simulink model "CML_Static_Sensory_Weighting"  (R2015a)
settings: Solver=ode4  SolverMode=MultiTasking  StartTime=0.0  StopTime=inf  FixedStep=BKIN_STEP_TIME  RelTol=1e-3
StartFcn:
  |  warndlg('Dexterit-E models cannot run under simulation. Please compile your model and run it from within Dexterit-E.');set_param(bdroot,'SimulationCommand','stop')
model workspace (MAT data in the model file):
  col_x = 1
  col_y = 2
  RADIUS_VIS = 3
  DELAY_POST_TRIAL_COL = 14
  BKIN_STEP_TIME = 0.00025
  START_WAIT_TIME_COL = 8
  E_START_TRIAL = 2
  E_START_REACHED = 4
  E_GO_CUE = 14
  E_MOVE_TIMEOUT = 21
  E_END_TRIAL = 20
  STROKE_WIDTH = 5
  K_HOLDTIME = 2
  K_ROBOT_RAMP_TIME = 3
  E_ROBOT_RETURN_TO_START = 10
  E_ENABLED_CONTROLLER = 31
  K_TIME_TO_START = 4
  E_HOLD_POS = 12
  BKIN_KINEMATIC_FRAME_SIZE = 400
  E_NO_EVENT = 0
  CP1 = 15
  CP2 = 16
  CP3 = 17
  CP4 = 18
  MOVE_TO_REF_TIME = 9
  REPOSITION_TIME = 11
  TRIAL_TYPE = 1
  E_RESPONSE_RECORDED = 18
  REPORT_TIME = 13
  REF_COLOR = 4
  START_TARGET_COL = 2
  REF_TARGET_COL = 3
  REF_HOLD_TIME = 10
  WAIT_REPORT_TIME = 12
  K_VEL_MIN = 1
  E_HAND_MOVING = 16
  E_MOVING_TO_REF = 6
  E_WAIT_AT_REF = 8
  TEXT1 = 6
  TEXT2 = 7
  TEXT3 = 8
  K_CUE_TARGET = 5
  E_START_REACHED2 = 5
  TEXT4 = 9
  CONTINUE = 4
  E_PAUSE = 40
  K_XJITTER = 6
  K_YJITTER = 7
  K_REF_START_TARGET = 8
  VY_TARG_OFFSET = 4
  PY_TARG_OFFSET = 5
  VX_TARG_OFFSET = 6
  PX_TARG_OFFSET = 7
libraries: Video x8, slrtlib x4, General x3, KINARM_general x2, KINARM_loads x2, xpcnilib x1
CloseFcn:
  | rtwprivate ssgencode ModelCloseRequest b2lab2d
settings Model: ModifiedComment=chris -- Wed Feb 16 09:18:30 2005 -- Version 1.1384  ModifiedHistory=Feb 16/05 - Add error repeat, add offset ramp  ExtModeArmWhenConnect=off  ExtModeLogAll=off  Creator=Chris Grebeldinger  LastModifiedBy=User
settings SolverCC: EnableConcurrentExecution=on  AutoInsertRateTranBlk=on
settings DataIOCC: LimitDataPoints=off  SignalLoggingSaveFormat=ModelDataLogs  SaveOutput=off  SaveTime=off  SignalLoggingName=sigsOut
settings OptimizationCC: BlockReduction=off  BooleanDataType=off  OptimizeBlockIOStorage=off  BufferReuse=off  GlobalBufferReuse=off  ExpressionFolding=off  ExpressionDepthLimit=2147483647  LocalBlockOutputs=off  InitFltsAndDblsToZero=on
settings DebuggingCC: SaveWithParameterizedLinksMsg=none  UnderspecifiedInitializationDetection=Classic  MergeDetectMultiDrivingBlocksExec=none  SignalResolutionControl=TryResolveAllWithWarning  MultiTaskDSMMsg=warning  FcnCallInpInsideContextMsg=UseLocalSettings  StateNameClashWarn=warning  StrictBusMsg=ErrorOnBusTreatedAsVector
settings HardwareCC: ProdIntDivRoundTo=Zero  ProdEndianess=LittleEndian  ProdLongLongMode=on  ProdHWDeviceType=Generic->32-bit x86 compatible  TargetHWDeviceType=32-bit Generic
settings SFSimCC: SimCustomHeaderCode="#include \"stdlib.h\""  SFSimEcho=off  SimParseCustomCode=off
settings RTWCC: SystemTargetFile=slrt.tlc  TemplateMakefile=slrt_default_tmf  Description=Simulink Real-Time  CustomSourceCode="#include \"stdlib.h\""
settings CodeAppCC: MaxIdLength=63
settings SimulinkRealTimeCC: TargetFcnLib=ansi_tfl_tmw.mat  GeneratePreprocessorConditionals=Disable all  xPCisDownloadable=off  xPCisDefaultEnv=off

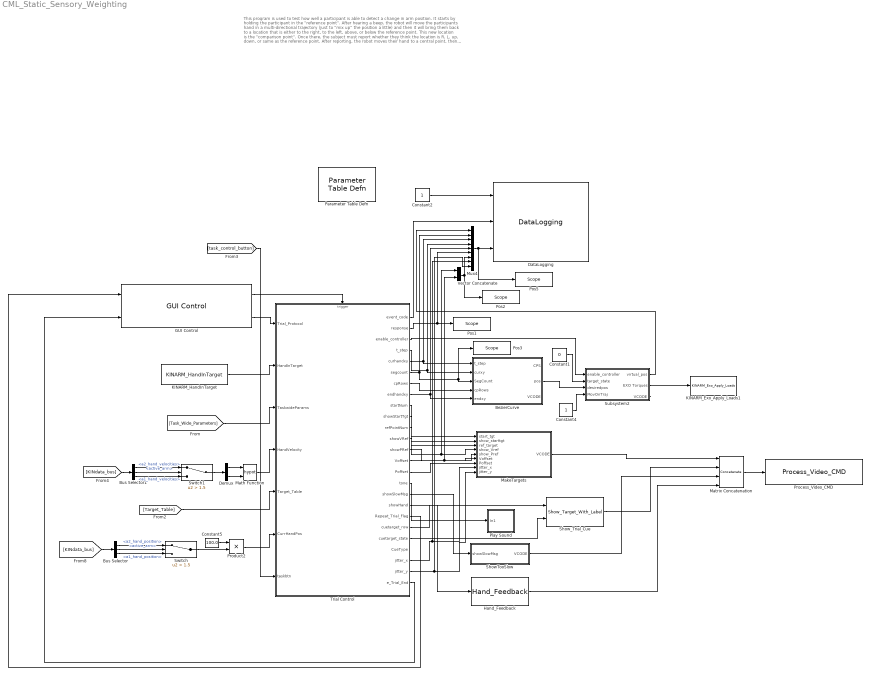
== system CML_Static_Sensory_Weighting ==
  note: This program is used to test how well a participant is able to detect a change in arm position.
      | It starts by holding the participant in the "reference point". After hearing a beep, the robot
      | will move the participants hand in a multi-directional trajectory (just to "mix up" the position a little)
      | and then it will bring them back to a location that is either to the right, to the left, above, or below
      | the reference point. This new location is the "comparison point". Once there, the subject must
      | report whether they think the location is R, L, up, down, or same as the reference point. After
      | reporting, the robot moves their hand to a central point, then back to the reference point to begin
      | the next trial.
      | A staircase updates for each direction, until a direction's staircase experiences 3 duirection
      | reversals in 6 trials, or 25 repetitions.
  BezierCurve : Subsystem
  Bus Selector : BusSelector  OutputSignals=Robot2.a2_hand_position,KINDataGeneral.active_arm,Robot1.a1_hand_position
  Bus Selector1 : BusSelector  OutputSignals=Robot2.a2_hand_velocities,KINDataGeneral.active_arm,Robot1.a1_hand_velocities
  Constant1 : Constant  Value=0
  Constant2 : Constant
  Constant4 : Constant
  Constant5 : Constant  Value=100.0
  DataLogging : General/DataLogging  log_event_codes=on  log_analog_inputs=on  show_time_remaining=off  ecat_include=on
  Demux : Demux  Outputs=2
  GUI Control : General/GUI Control  task_version=1.0  show_repeat_trial_flag=on  use_custom_tp=off  target_type_str=Circle  Target_Type=1  XYcols=[1 2]  Vcols=3  Lcols=4  indices_padding=[0 0 0 0;0 0 0 0]  target_table_rows=64  load_table_rows=20  tp_table_rows=100
  Hand_Feedback : KINARM_general/Hand_Feedback  feedback_cntl_src=status only
  KINARM_Exo_Apply_Loads1 : KINARM_loads/KINARM_Exo_Apply_Loads  up_duration=500  down_duration=500  max_torque=8  limit_motors=off
  KINARM_HandInTarget : KINARM_general/KINARM_HandInTarget  use_dominant_hand=on  target_type=Circle  num_states=1  attribcol1=[RADIUS_VIS]  attribcol2=[0]  attribcol3=[0]  attribcol4=[0]  attribcol5=[0]
  MakeTargets : Subsystem
  Math Function : Math  Operator=hypot  SaturateOnIntegerOverflow=on
  Matrix Concatenation : Concatenate  NumInputs=4  Mode=Multidimensional array
  Mux4 : Mux  Inputs=9
  Parameter Table Defn : General/Parameter Table Defn  ShowInLibBrowser=0
  Play Sound : Subsystem
  Pos1 : slrtlib/Displays and Logging/Scope   scopeno=2  scopetype=Target  autostart=on  viewmode=Numerical  formatstr='%15.6f'  grid=on  ylimits=[-10,10]  nosamples=250  noprepostsamples=0  interleave=1  triggermode=FreeRun  triggersignal=1  trigsignalfromport=off  triggerlevel=0.0  triggerslope=Either  triggerscope=1  triggersample=0  filename=data.dat  mode=Lazy  writesize=512  autorestart=off  dynamicfilemode=off  maxwritefilesize=512*1024^2
  Pos2 : slrtlib/Displays and Logging/Scope   scopeno=3  scopetype=Target  autostart=on  viewmode=Numerical  formatstr='%15.6f'  grid=on  ylimits=[-10,10]  nosamples=250  noprepostsamples=0  interleave=1  triggermode=FreeRun  triggersignal=1  trigsignalfromport=off  triggerlevel=0.0  triggerslope=Either  triggerscope=1  triggersample=0  filename=data.dat  mode=Lazy  writesize=512  autorestart=off  dynamicfilemode=off  maxwritefilesize=512*1024^2
  Pos3 : slrtlib/Displays and Logging/Scope   scopeno=4  scopetype=Target  autostart=on  viewmode=Numerical  formatstr='%15.6f'  grid=on  ylimits=[-10,10]  nosamples=250  noprepostsamples=0  interleave=1  triggermode=FreeRun  triggersignal=1  trigsignalfromport=off  triggerlevel=0.0  triggerslope=Either  triggerscope=1  triggersample=0  filename=data.dat  mode=Lazy  writesize=512  autorestart=off  dynamicfilemode=off  maxwritefilesize=512*1024^2
  Pos5 : slrtlib/Displays and Logging/Scope   scopeno=1  scopetype=Target  autostart=on  viewmode=Numerical  formatstr='%15.6f'  grid=on  ylimits=[-10,10]  nosamples=250  noprepostsamples=0  interleave=1  triggermode=FreeRun  triggersignal=1  trigsignalfromport=off  triggerlevel=0.0  triggerslope=Either  triggerscope=1  triggersample=0  filename=data.dat  mode=Lazy  writesize=512  autorestart=off  dynamicfilemode=off  maxwritefilesize=512*1024^2
  Process_Video_CMD : Video/Process_Video_CMD  video_delay=50
  Product2 : Product
  ShowTooSlow : Subsystem
  Show_Trial_Cue : Video/Show_Target_With_Label  target_type=Circle  num_states=4  attribcol1=[0 0 0 RADIUS_VIS TEXT1 REF_COLOR STROKE_WIDTH]  attribcol2=[0 0 0 RADIUS_VIS TEXT2 REF_COLOR STROKE_WIDTH]  attribcol3=[0 0 0 RADIUS_VIS TEXT3 REF_COLOR STROKE_WIDTH]  attribcol4=[0 0 0 RADIUS_VIS TEXT4 REF_COLOR STROKE_WIDTH]  attribcol5=[0 0 0 0 0 0 0]  stateindices_padding=[0 0 0 0;0 0 0 0;0 0 0 0;0 0 0 0;0 0 0 0]  source=dialog  opacity=100  target_display=Both subject and operator displays
  Subsystem2 : Subsystem
  Switch : Switch  Criteria=u2 > Threshold  Threshold=1.5
  Switch1 : Switch  Criteria=u2 > Threshold  Threshold=1.5
  Trial Control : Stateflow chart  TreatAsAtomicUnit=on
  Vector Concatenate : Concatenate
  wires:
  [Task_Wide_Parameters] -> Trial Control/3(TaskwideParams)
  Trial Control/1(event_code) -> DataLogging/2
  [KINdata_bus] -> Bus Selector1/1
  GUI Control/2 -> Trial Control/1(Trial_Protocol)
  Trial Control/7(cpRows) -> BezierCurve/4(cpRows)
  Trial Control/5(curhandxy) -> Mux4/4, BezierCurve/2(curxy)
  Trial Control/6(segcount) -> Pos3/1, BezierCurve/3(SegCount), Mux4/2
  Trial Control/4(t_step) -> BezierCurve/1(t_step), Mux4/3
  Trial Control/11(refPointNum) -> MakeTargets/3(ref_target)
  BezierCurve/2(pos) -> Subsystem2/3(desiredpos)
  KINARM_HandInTarget/1 -> Trial Control/2(HandInTarget)
  Trial Control/8(endhandxy) -> BezierCurve/5("endxy "), Mux4/5
  Trial Control/16(tone) -> Play Sound/1(In1)
  [Target_Table] -> Trial Control/5(Target_Table)
  Trial Control/19(Repeat_Trial_Flag) -> GUI Control/1
  Mux4/1 -> Pos5/1, DataLogging/3
  Constant2/1 -> DataLogging/1
  Subsystem2/2(EXO Torques) -> KINARM_Exo_Apply_Loads1/1
  Trial Control/25(e_Trial_End) -> GUI Control/2
  Subsystem2/3(VCODE) -> ?
  Subsystem2/1(virtual_pos) -> Mux4/1
  Constant4/1 -> Subsystem2/4(MovOnTraj)
  Trial Control/3(enable_controller) -> Subsystem2/1(enable_controller)
  [KINdata_bus] -> Bus Selector/1
  Bus Selector/2 -> Switch/2  "<active_arm>"
  Bus Selector/1 -> Switch/1  "<a2_hand_position>"
  Bus Selector/3 -> Switch/3  "<a1_hand_position>"
  Switch/1 -> Product2/2
  Constant5/1 -> Product2/1
  Product2/1 -> Trial Control/6(CurrHandPos)
  MakeTargets/1(VCODE) -> Matrix Concatenation/1
  Trial Control/2(response) -> Mux4/6, Pos1/1
  Trial Control/18(showHand) -> Hand_Feedback/1
  Hand_Feedback/1 -> Matrix Concatenation/4
  Trial Control/14(Voffset) -> MakeTargets/6(Voffset)
  Trial Control/15(Poffset) -> MakeTargets/7(Poffset)
  Trial Control/9(startNum) -> MakeTargets/1(start_tgt)
  Trial Control/10(showStartTgt) -> MakeTargets/2(show_starttgt)
  Vector Concatenate/1 -> Pos2/1, Mux4/7
  Trial Control/12(showVRef) -> Vector Concatenate/1, MakeTargets/4(show_Vref)
  Trial Control/13(showPRef) -> Vector Concatenate/2, MakeTargets/5(show_Pref)
  Bus Selector1/2 -> Switch1/2  "<active_arm>"
  Bus Selector1/1 -> Switch1/1  "<a2_hand_velocities>"
  Bus Selector1/3 -> Switch1/3  "<a1_hand_velocities>"
  Math Function/1 -> Trial Control/4(HandVelocity)
  Switch1/1 -> Demux/1
  Demux/1 -> Math Function/1
  Demux/2 -> Math Function/2
  Trial Control/17(showSlowMsg) -> ShowTooSlow/1(showSlowMsg)
  ShowTooSlow/1(VCODE) -> Matrix Concatenation/3
  Constant1/1 -> Subsystem2/2(target_state)
  Trial Control/20(cuetarget_row) -> Show_Trial_Cue/1
  Trial Control/21(cuetarget_state) -> Show_Trial_Cue/2
  Show_Trial_Cue/1 -> Matrix Concatenation/2
  [task_control_button] -> Trial Control/7(taskbtn)
  GUI Control/1 -> Trial Control/Trigger
  Trial Control/23(jitter_x) -> Mux4/8, MakeTargets/8("jitter_x ")
  Trial Control/24(jitter_y) -> Mux4/9, MakeTargets/9("jitter_y ")
  Matrix Concatenation/1 -> Process_Video_CMD/1

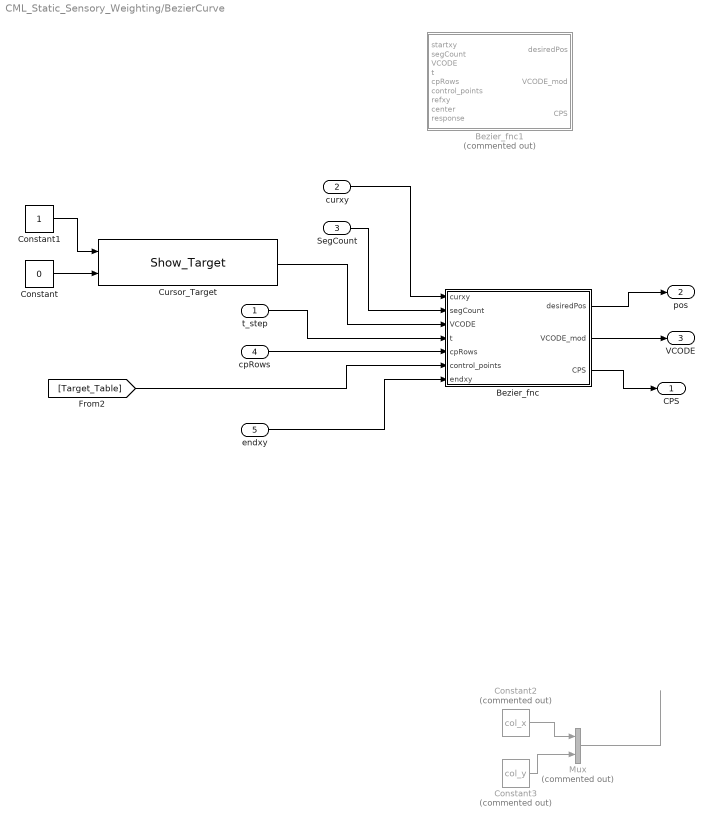
== system CML_Static_Sensory_Weighting/BezierCurve ==
  t_step : Inport  PortDimensions=1
  curxy : Inport  Port=2  PortDimensions=[1 2]
  SegCount : Inport  Port=3  PortDimensions=1
  cpRows : Inport  Port=4  PortDimensions=[1 5]
  "endxy " : Inport  Port=5  PortDimensions=[1 2]
  Bezier_fnc : MATLAB Function  TreatAsAtomicUnit=on
  Bezier_fnc1 : MATLAB Function  Commented=on  TreatAsAtomicUnit=on
  Constant : Constant  Value=0
  Constant1 : Constant
  Constant2 : Constant  Commented=on  Value=col_x
  Constant3 : Constant  Commented=on  Value=col_y
  Cursor_Target : Video/Show_Target  target_type=Circle  num_states=1  attribcol1=[REF_COLOR 0 0 RADIUS_VIS]  attribcol2=[0 0 0 0]  attribcol3=[0 0 0 0]  attribcol4=[0 0 0 0]  attribcol5=[0 0 0 0]  stateindices_padding=[0 0 0 0 0 0 0;0 0 0 0 0 0 0;0 0 0 0 0 0 0;0 0 0 0 0 0 0;0 0 0 0 0 0 0]  source=dialog  opacity=100  target_display=Both subject and operator displays  num_col=4
  Mux : Mux  Commented=on  Inputs=2
  CPS : Outport  PortDimensions=[1 8]
  pos : Outport  Port=2  OutDataTypeStr=double  PortDimensions=[1 2]
  VCODE : Outport  Port=3
  wires:
  Cursor_Target/1 -> Bezier_fnc/3(VCODE)
  Bezier_fnc/2(VCODE_mod) -> VCODE/1
  [Target_Table] -> Bezier_fnc/6(control_points)
  Bezier_fnc/1(desiredPos) -> pos/1
  Constant1/1 -> Cursor_Target/1
  curxy/1 -> Bezier_fnc/1(curxy)
  SegCount/1 -> Bezier_fnc/2(segCount)
  cpRows/1 -> Bezier_fnc/5(cpRows)
  "endxy "/1 -> Bezier_fnc/7(endxy)
  Constant/1 -> Cursor_Target/2
  t_step/1 -> Bezier_fnc/4(t)
  Mux/1 -> ?
  Constant2/1 -> Mux/1
  Constant3/1 -> Mux/2
  Bezier_fnc/3(CPS) -> CPS/1

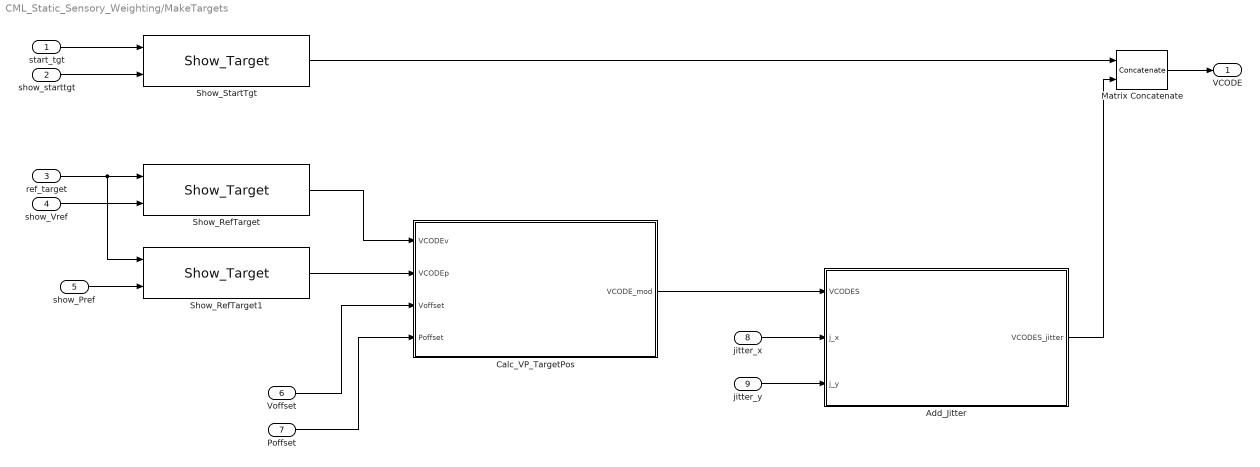
== system CML_Static_Sensory_Weighting/MakeTargets ==
  start_tgt : Inport
  show_starttgt : Inport  Port=2
  ref_target : Inport  Port=3
  show_Vref : Inport  Port=4
  show_Pref : Inport  Port=5
  Voffset : Inport  Port=6
  Poffset : Inport  Port=7
  "jitter_x " : Inport  Port=8
  "jitter_y " : Inport  Port=9
  Add_Jitter : MATLAB Function  TreatAsAtomicUnit=on
  Calc_VP_TargetPos : MATLAB Function  TreatAsAtomicUnit=on
  Matrix Concatenate : Concatenate  Mode=Multidimensional array
  Show_RefTarget : Video/Show_Target  target_type=Circle  num_states=1  attribcol1=[REF_COLOR 0 0 RADIUS_VIS]  attribcol2=[0 0 0 0]  attribcol3=[0 0 0 0]  attribcol4=[0 0 0 0]  attribcol5=[0 0 0 0]  stateindices_padding=[0 0 0 0 0 0 0;0 0 0 0 0 0 0;0 0 0 0 0 0 0;0 0 0 0 0 0 0;0 0 0 0 0 0 0]  source=dialog  opacity=100  target_display=Both subject and operator displays  num_col=4
  Show_RefTarget1 : Video/Show_Target  target_type=Circle  num_states=1  attribcol1=[REF_COLOR 0 0 RADIUS_VIS]  attribcol2=[0 0 0 0]  attribcol3=[0 0 0 0]  attribcol4=[0 0 0 0]  attribcol5=[0 0 0 0]  stateindices_padding=[0 0 0 0 0 0 0;0 0 0 0 0 0 0;0 0 0 0 0 0 0;0 0 0 0 0 0 0;0 0 0 0 0 0 0]  source=dialog  opacity=100  target_display=Both subject and operator displays  num_col=4
  Show_StartTgt : Video/Show_Target  target_type=Circle  num_states=1  attribcol1=[REF_COLOR 0 0 RADIUS_VIS]  attribcol2=[0 0 0 0]  attribcol3=[0 0 0 0]  attribcol4=[0 0 0 0]  attribcol5=[0 0 0 0]  stateindices_padding=[0 0 0 0 0 0 0;0 0 0 0 0 0 0;0 0 0 0 0 0 0;0 0 0 0 0 0 0;0 0 0 0 0 0 0]  source=dialog  opacity=100  target_display=Both subject and operator displays  num_col=4
  VCODE : Outport
  wires:
  ref_target/1 -> Show_RefTarget1/1, Show_RefTarget/1
  show_Vref/1 -> Show_RefTarget/2
  Show_RefTarget/1 -> Calc_VP_TargetPos/1(VCODEv)
  Voffset/1 -> Calc_VP_TargetPos/3(Voffset)
  Poffset/1 -> Calc_VP_TargetPos/4(Poffset)
  Calc_VP_TargetPos/1(VCODE_mod) -> Add_Jitter/1(VCODES)
  start_tgt/1 -> Show_StartTgt/1
  show_starttgt/1 -> Show_StartTgt/2
  Matrix Concatenate/1 -> VCODE/1
  Show_StartTgt/1 -> Matrix Concatenate/1
  show_Pref/1 -> Show_RefTarget1/2
  Show_RefTarget1/1 -> Calc_VP_TargetPos/2(VCODEp)
  Add_Jitter/1(VCODES_jitter) -> Matrix Concatenate/2
  "jitter_x "/1 -> Add_Jitter/2(j_x)
  "jitter_y "/1 -> Add_Jitter/3(j_y)

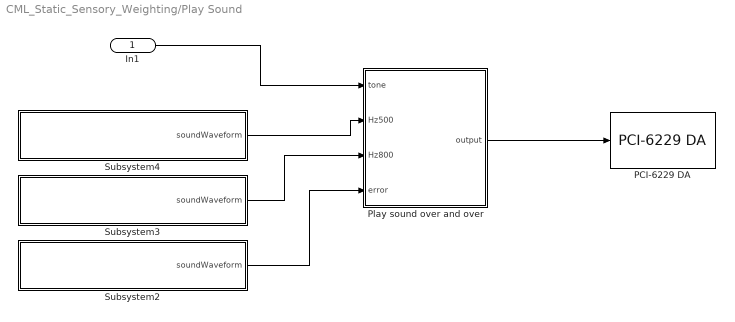
== system CML_Static_Sensory_Weighting/Play Sound ==
  In1 : Inport
  PCI-6229 DA : xpcnilib/D//A/M Series/PCI-6229 DA  channel=[1]  reset=[1]  initValue=[0]  sampletime=-1  slot=-1
  Play sound over and over : MATLAB Function  TreatAsAtomicUnit=on
  Subsystem2 : Subsystem  mask(Load Waveform Into Variable){fileName=errorbeep.mat}
      mask prompts: fileName "Name of .mat Data File (must be in current directory)"
      mask help: This block will load the .MAT file specified in the dialog, and put the first variable into a GoTo called 'soundWaveform'.
      mask init:
      | filenameFromMask = get_param(gcb, 'fileName');
      | 
      | try 
      | 	dataFromFile = load(filenameFromMask);
      | 	names = fieldnames(dataFromFile);
      | 	soundDataFromFile = dataFromFile.(names{1});
      | 	display(['Sound waveform from file ''' filenameFromMask ''' loaded.']);
      | catch ME
      | 	display(ME.message)
      | end
      mask Help:
      | Enter the name a .MAT file containing a single vector or matrix. The .MAT file must be located in the current directory.
      | 
      | The first variable from the .MAT file will be put into a Goto called 'soundWaveform'.
      mask Display: disp(['Load waveform from ''' filenameFromMask ''''])
  Subsystem3 : Subsystem  mask(Load Waveform Into Variable){fileName=Hz800}
      mask prompts: fileName "Name of .mat Data File (must be in current directory)"
      mask help: This block will load the .MAT file specified in the dialog, and put the first variable into a GoTo called 'soundWaveform'.
      mask init: same as CML_Static_Sensory_Weighting/Play Sound/Subsystem2
      mask Help:
      | Enter the name a .MAT file containing a single vector or matrix. The .MAT file must be located in the current directory.
      | 
      | The first variable from the .MAT file will be put into a Goto called 'soundWaveform'.
      mask Display: disp(['Load waveform from ''' filenameFromMask ''''])
  Subsystem4 : Subsystem  mask(Load Waveform Into Variable){fileName=Hz500}
      mask prompts: fileName "Name of .mat Data File (must be in current directory)"
      mask help: This block will load the .MAT file specified in the dialog, and put the first variable into a GoTo called 'soundWaveform'.
      mask init: same as CML_Static_Sensory_Weighting/Play Sound/Subsystem2
      mask Help:
      | Enter the name a .MAT file containing a single vector or matrix. The .MAT file must be located in the current directory.
      | 
      | The first variable from the .MAT file will be put into a Goto called 'soundWaveform'.
      mask Display: disp(['Load waveform from ''' filenameFromMask ''''])
  wires:
  Play sound over and over/1(output) -> PCI-6229 DA/1
  Subsystem3/1(soundWaveform) -> Play sound over and over/3(Hz800)
  Subsystem4/1(soundWaveform) -> Play sound over and over/2(Hz500)
  In1/1 -> Play sound over and over/1(tone)
  Subsystem2/1(soundWaveform) -> Play sound over and over/4(error)

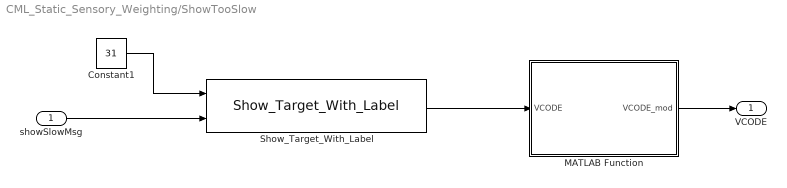
== system CML_Static_Sensory_Weighting/ShowTooSlow ==
  showSlowMsg : Inport
  Constant1 : Constant  Value=31
  MATLAB Function : MATLAB Function  TreatAsAtomicUnit=on
  Show_Target_With_Label : Video/Show_Target_With_Label  target_type=Circle  num_states=1  attribcol1=[0 0 0 RADIUS_VIS 0 REF_COLOR RADIUS_VIS]  attribcol2=[0 0 0 0 0 0 0]  attribcol3=[0 0 0 0 0 0 0]  attribcol4=[0 0 0 0 0 0 0]  attribcol5=[0 0 0 0 0 0 0]  stateindices_padding=[0 0 0 0;0 0 0 0;0 0 0 0;0 0 0 0;0 0 0 0]  source=dialog  opacity=100  target_display=Both subject and operator displays
  VCODE : Outport
  wires:
  showSlowMsg/1 -> Show_Target_With_Label/2
  Constant1/1 -> Show_Target_With_Label/1
  Show_Target_With_Label/1 -> MATLAB Function/1(VCODE)
  MATLAB Function/1(VCODE_mod) -> VCODE/1

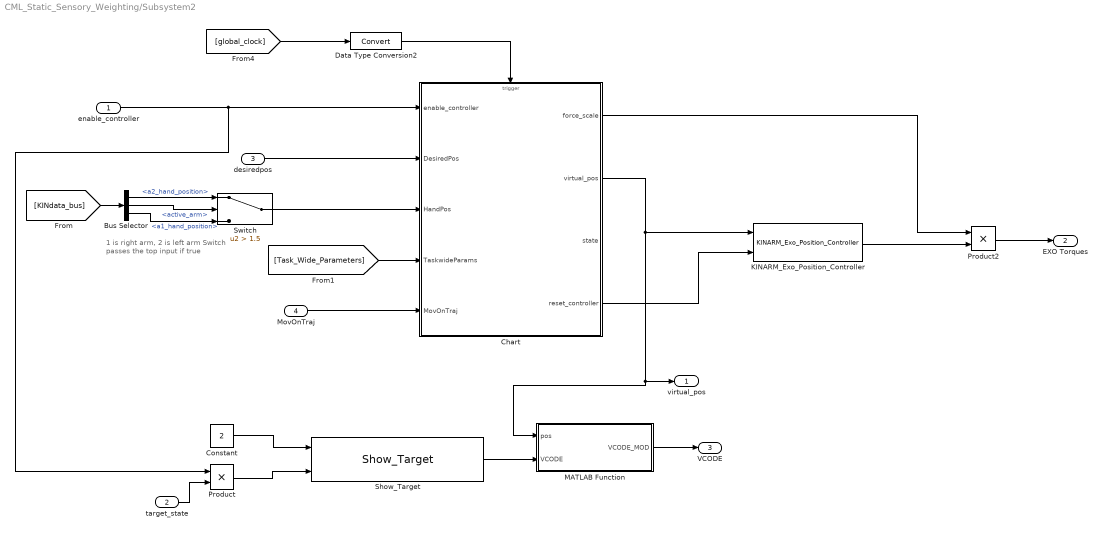
== system CML_Static_Sensory_Weighting/Subsystem2 ==
  note: 1 is right arm, 2 is left arm
      | Switch passes the top input if true
  enable_controller : Inport
  target_state : Inport  Port=2
  desiredpos : Inport  Port=3
  MovOnTraj : Inport  Port=4
  Bus Selector : BusSelector  OutputSignals=Robot2.a2_hand_position,KINDataGeneral.active_arm,Robot1.a1_hand_position
  Chart : Stateflow chart  TreatAsAtomicUnit=on
  Constant : Constant  Value=2
  Data Type Conversion2 : DataTypeConversion
  KINARM_Exo_Position_Controller : KINARM_loads/KINARM_Exo_Position_Controller  use_dom_hand=on  KINARM_Type=Human  inertias_for_FF=KINARM robot & arm troughs & subject  angles_or_XY=End-point (global x/y)  sample_time=0.001
  MATLAB Function : MATLAB Function  TreatAsAtomicUnit=on
  Product : Product
  Product2 : Product
  Show_Target : Video/Show_Target  target_type=Circle  num_states=1  attribcol1=[REF_COLOR 0 0 RADIUS_VIS]  attribcol2=[0 0 0 0]  attribcol3=[0 0 0 0]  attribcol4=[0 0 0 0]  attribcol5=[0 0 0 0]  stateindices_padding=[0 0 0 0 0 0 0;0 0 0 0 0 0 0;0 0 0 0 0 0 0;0 0 0 0 0 0 0;0 0 0 0 0 0 0]  source=dialog  opacity=100  target_display=Both subject and operator displays  num_col=4
  Switch : Switch  Criteria=u2 > Threshold  Threshold=1.5
  virtual_pos : Outport
  EXO Torques : Outport  Port=2
  VCODE : Outport  Port=3
  wires:
  [KINdata_bus] -> Bus Selector/1
  Bus Selector/2 -> Switch/2  "<active_arm>"
  [Task_Wide_Parameters] -> Chart/4(TaskwideParams)
  [global_clock] -> Data Type Conversion2/1
  Data Type Conversion2/1 -> Chart/Trigger
  Chart/2(virtual_pos) -> MATLAB Function/1(pos), virtual_pos/1, KINARM_Exo_Position_Controller/1
  MovOnTraj/1 -> Chart/5(MovOnTraj)
  Switch/1 -> Chart/3(HandPos)
  desiredpos/1 -> Chart/2(DesiredPos)
  Constant/1 -> Show_Target/1
  Show_Target/1 -> MATLAB Function/2(VCODE)
  MATLAB Function/1(VCODE_MOD) -> VCODE/1
  KINARM_Exo_Position_Controller/1 -> Product2/2
  Product2/1 -> EXO Torques/1
  Chart/1(force_scale) -> Product2/1
  Chart/4(reset_controller) -> KINARM_Exo_Position_Controller/2
  Bus Selector/1 -> Switch/1  "<a2_hand_position>"
  Bus Selector/3 -> Switch/3  "<a1_hand_position>"
  enable_controller/1 -> Product/1, Chart/1(enable_controller)
  Product/1 -> Show_Target/2
  target_state/1 -> Product/2

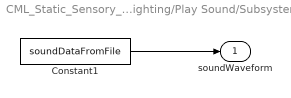
== system CML_Static_Sensory_Weighting/Play Sound/Subsystem2 ==
  Constant1 : Constant  Value=soundDataFromFile  VectorParams1D=off  SampleTime=-1
  soundWaveform : Outport
  wires:
  Constant1/1 -> soundWaveform/1

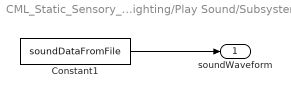
== system CML_Static_Sensory_Weighting/Play Sound/Subsystem3 ==
  Constant1 : Constant  Value=soundDataFromFile
  soundWaveform : Outport
  wires:
  Constant1/1 -> soundWaveform/1

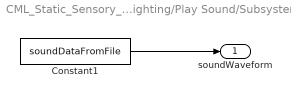
== system CML_Static_Sensory_Weighting/Play Sound/Subsystem4 ==
  Constant1 : Constant  Value=soundDataFromFile
  soundWaveform : Outport
  wires:
  Constant1/1 -> soundWaveform/1

== matlab function CML_Static_Sensory_Weighting/BezierCurve/Bezier_fnc1 ==
  data: startxy input size=[1 2]; segCount input; desiredPos output size=[1 2]; VCODE input; VCODE_mod output; t input; cpRows input size=[1 5]; control_points input; refxy input size=[1 2]; CPS output size=[1 8]; center input; response input
function [desiredPos,VCODE_mod, CPS] = fcn(startxy,segCount,VCODE,t,cpRows,control_points,refxy,center,response)
%#codegen

VCODE_mod = VCODE;

%clip t just in case!
if t < 0
    t = 0;
elseif t > 1;
    t = 1;
end

t = t-sin(2*pi*t)/(2*pi);  %use the bell-shaped velocity profile from the trajectory controller

dPos = [0 0];
cp1 = [0 0];
cp2 = [0 0];
cp3 = [0 0];
cp4 = [0 0];
cp5 = [0 0];
cp6 = [0 0];

% first seg is always used to get the hand to the next trial's reference
if segCount == 1
        %6 point bezier
    cp1 = startxy;
    cp2 = [control_points(cpRows(1),1), control_points(cpRows(1),2)]; %CP1X and CP1Y
    cp3 = [control_points(cpRows(2),1), control_points(cpRows(2),2)]; %CP2X and CP2Y
    cp4 = [control_points(cpRows(3),1), control_points(cpRows(3),2)]; %CP3X and CP3Y
    cp5 = [control_points(cpRows(4),1), control_points(cpRows(4),2)]; %CP4X and CP4Y %+startxy(1)-center(1)+startxy(2)-center(2)
    cp6 = refxy;
    
    dPos = ((1-t)^5)*cp1 + 5*t*((1-t)^4)*cp2 + 10*(t^2)*((1-t)^3)*cp3 + 10*(t^3)*((1-t)^2)*cp4 + 5*(t^4)*(1-t)*cp5 + (t^5)*cp6;

    

elseif segCount == 2 
        %6 point bezier
    cp1 = refxy;
    cp2 = [control_points(cpRows(1),1), control_points(cpRows(1),2)]; %CP1X and CP1Y
    cp3 = [control_points(cpRows(2),1), control_points(cpRows(2),2)]; %CP2X and CP2Y
    cp4 = [control_points(cpRows(3),1), control_points(cpRows(3),2)]; %CP3X and CP3Y
    cp5 = [control_points(cpRows(4),1), control_points(cpRows(4),2)]; %CP4X and CP4Y
    cp6 = startxy;
    
    dPos = ((1-t)^5)*cp1 + 5*t*((1-t)^4)*cp2 + 10*(t^2)*((1-t)^3)*cp3 + 10*(t^3)*((1-t)^2)*cp4 + 5*(t^4)*(1-t)*cp5 + (t^5)*cp6;

elseif segCount == 3
    %hold still where the subject is currently (after reporting)
    cp1 = response; 
    cp2 = [NaN NaN];
    cp3 = [NaN NaN];
    cp4 = [NaN NaN];
    cp5 = [NaN NaN];
    
    dPos = cp1;
    
elseif segCount == 4
    %linear bezier using origin and reference
    %point from the next trial
    cp1 = response;
    cp2 = startxy;
    cp3 = [NaN NaN];
    cp4 = [NaN NaN];
    cp5 = [NaN NaN];
    
    dPos = (1-t)*cp1 + t*cp2;
    
else    
    cp1 = [NaN NaN];
    cp2 = [NaN NaN];
    cp3 = [NaN NaN];
    cp4 = [NaN NaN];
    cp5 = [NaN NaN];
    
    dPos = startxy;
end



desiredPos = dPos; %to get to cm
desiredPos = desiredPos/100;

CPS = [cp2 cp3 cp4 cp5];

VCODE_mod(3) = desiredPos(1); %convert to meters
VCODE_mod(4) = desiredPos(2); %convert to meters

% elseif segCount == 3 
%     %cubic ends at compPoint
%     cp1 = [control_points(cpRows(3),1), control_points(cpRows(3),2)];
%     cp2 = [control_points(cpRows(4),1), control_points(cpRows(4),2)]; %CP4X and CP4Y
%     cp3 = [control_points(cpRows(5),1), control_points(cpRows(5),2)];
%     cp4 = compPoint;
%     
%     dPos = ((1-t)^3)*cp1 + 3*((1-t)^2)*t*cp2 + 3*(1-t)*(t^2)*cp3 + (t^3)*cp4;

== matlab function CML_Static_Sensory_Weighting/ShowTooSlow/MATLAB Function ==
  data: VCODE input; VCODE_mod output
function VCODE_mod = fcn(VCODE)
%#codegen

VCODE_mod = VCODE;

textout = double('Too Slow');

VCODE_mod(1,15:min([15+length(textout)-1,64])) = textout(1:min([length(textout),50])); %write out as many the characters as possible into the VCODE
VCODE_mod(1,min([15+length(textout)+1,64])) = 0;  %terminate the string!

== matlab function CML_Static_Sensory_Weighting/MakeTargets/Calc_VP_TargetPos ==
  data: VCODEv input; VCODE_mod output; VCODEp input; Voffset input; Poffset input
function VCODE_mod = Calc_TargetPos(VCODEv,VCODEp,Voffset,Poffset)
%#codegen

VCODE_mod = [VCODEv; VCODEp; VCODEv];


%convert from cm to m
Voffset = Voffset/100;
Poffset = Poffset/100;

VCODE_mod(1,3) = VCODE_mod(1,3) + Voffset(1);  %V target
VCODE_mod(1,4) = VCODE_mod(1,4) + Voffset(2);  %V target
%Venable already set.
%if VCODE_mod(1,2) == 0  %If it's off, we'll set it to show on the operator screen only
%    VCODE_mod(1,2) = 3;
%end


VCODE_mod(2,3) = VCODE_mod(2,3) + Poffset(1);  %P target
VCODE_mod(2,4) = VCODE_mod(2,4) + Poffset(2);  %P target
%Penable already set
%VCODE_mod(2,2) = Penable;
% if Venable > 0  %If it's off, we'll set it to show on the operator screen only
%     VCODE_mod(2,2) = 3;
% end

VCODE_mod(3,2) = 3;  %actual ref target - show on screen only
VCODE_mod(3,5) = createcolor(0,0,100);



end





function color_value = createcolor(red, green, blue)
% CREATE_COLOR Given percentages of red, green and blue creates an RGB color.
% c = CREATE_COLOR(0, 100, 0) creates a pure green
% c = CREATE_COLOR(20, 0, 20) creates a dark magenta.

    red = bound(red);
    green = bound(green);
    blue = bound(blue);
    
    %convert to RGB bytes
    r = uint32(255 * (red / 100));
    g = uint32(255 * (green / 100));
    b = uint32(255 * (blue / 100));
    
    color_value = bitshift(r, 16) + bitshift(g, 8) + b;
    
end


function color = bound(c)
color = c;
if color < 0 || color > 100
    warning 'Valid values are 0-100'
    if color < 0
        color = 0;
    else
        color = 100;
    end
end
end

== matlab function CML_Static_Sensory_Weighting/Play Sound/Play sound over and over ==
  data: tone input; output output; Hz500 input; Hz800 input; error input
function output = fcn(tone,Hz500,Hz800,error)
%#codegen

persistent t last_tone_state
if isempty(t), t = 0; end
if isempty(last_tone_state), last_tone_state = 0; end

trigger = last_tone_state ~= tone;
if trigger > 0
    last_tone_state = tone;
end

output = 0;		% default
if t == 0 && trigger > 0
	% start the playing of the sound.
	t = t + 1;
end

if tone == 1
    data = Hz500;
elseif tone == 2
    data = Hz800;
elseif tone == 3
    data = error;
else 
    t = 0;
    data = 0;
end

if t > 0
	output = data(t);
	if t == length(data)
		t = 0;
	else
		t = t + 1;
	end
end

== stateflow chart CML_Static_Sensory_Weighting/Trial Control ==
  state Initialize1/
    //Initialization state
    Repeat_Trial_Flag = 0;
    ramp_time = TaskwideParams[K_ROBOT_RAMP_TIME];
    enable_controller = 0;
    tone = 0;
    showVRef = 0;
    showPRef = 0;
    showHand = 0;
    refPointNum = 0;
    tickCount = START_WAIT_TIME_COL;
    segcount = 3;
    showStartTgt = 0
    showSlowMsg = 0;
    showHand = 0;
  state Task1
    state MoveToStart/
      event_code = E_START_TRIAL;
      cuetarget_row = TaskwideParams[K_CUE_TARGET];
      cuetarget_state=Trial_Protocol[TRIAL_TYPE];
      // set up jitter
      startTarget_ref = TaskwideParams[K_REF_START_TARGET];
      // this pulls the reference start target, compares it to the task start target
      // and gets jitter values which will be used for modifying other targets
      startNum = Trial_Protocol[START_TARGET_COL]
      jitter_x=Target_Table[startNum][1]-Target_Table[startTarget_ref][1];
      jitter_y=Target_Table[startNum][2]-Target_Table[startTarget_ref][2];
      curhandxy[1] = CurrHandPos[1];
      curhandxy[2] = CurrHandPos[2];
      segcount = 3; //Hold still
      tone = 0;
      startxy[1] = Target_Table[startNum][1]; //x pos for start point
      startxy[2] = Target_Table[startNum][2]; //y pos for start point
      showStartTgt = 1;
      response[1] = 0;
      response[2] = 0;
      showHand = 0; // show hand at start for 500 ms
      showSlowMsg = 0;
      showVRef = 0;
      showPRef = 0;
      Repeat_Trial_Flag = 0;
      endhandxy[1] = startxy[1];
      endhandxy[2] = startxy[2];
      segcount = 2; // seg 2 starts from curxy and ends on the endxy
      enable_controller = 1;
      t_step = 0;
      //increment t_step on each clock cycle
      during:
      on e_clk: t_step = t_step + (1.0/ TaskwideParams[K_TIME_TO_START]);
    state InitPauseTrial1/
      // Just want to pause for a little
      event_code = E_PAUSE;
    state PauseStart/
      event_code = E_START_REACHED;
      showHand = 1; // show hand at start for 500 ms
      tickCount = 500;
    state PauseStart2/
      event_code = E_START_REACHED2;
      showHand = 0;
      tickCount = START_WAIT_TIME_COL;
      segcount = 5;  //hold at startxy point
      curhandxy[1] = CurrHandPos[1];
      curhandxy[2] = CurrHandPos[2];
      segcount = 3;
    state HoldStart/
      tickCount = Trial_Protocol[MOVE_TO_REF_TIME];
    state waitBeforeReport1/
      showHand = 0;
      refPointNum = Trial_Protocol[REF_TARGET_COL];
      refxy[1] = Target_Table[refPointNum][1]+jitter_x; //x pos for ref point
      refxy[2] = Target_Table[refPointNum][2]+jitter_y; //y pos for ref point
      Voffset[1] = Trial_Protocol[VX_TARG_OFFSET];
      Poffset[1] = Trial_Protocol[PX_TARG_OFFSET];
      Voffset[2] = Trial_Protocol[VY_TARG_OFFSET];
      Poffset[2] = Trial_Protocol[PY_TARG_OFFSET];
    state Move2reference_seg1P/
      //from start, move to reference point
      event_code = E_MOVING_TO_REF;
      tickCount = Trial_Protocol[START_WAIT_TIME_COL] ;
      //start is startxy
      curhandxy[1] = CurrHandPos[1];
      curhandxy[2] = CurrHandPos[2];
      cpRows[1] = Trial_Protocol[CP1]; //CP1
      cpRows[2] = Trial_Protocol[CP2];
      cpRows[3] = -1;
      cpRows[4] = -1;//CP4
      endhandxy[1] = refxy[1] + Poffset[1];
      endhandxy[2] = refxy[2] + Poffset[2];
      t_step = 0;
      segcount = 1;  //move along curvy bezier curve
      //increment t_step on each clock cycle
      during:
      on e_clk: t_step = t_step + (1.0/ (Trial_Protocol[MOVE_TO_REF_TIME]));
    state ShowReference/
      //from origin, move to new reference point
      event_code = E_WAIT_AT_REF;
      tone = 1;
      showHand = 0;
      showVRef = 1;
      showPRef = 0;
      tickCount = Trial_Protocol[REF_HOLD_TIME] ; //MI this should be it's own time? 1200ms
    state BlankScreen/
      tickCount = Trial_Protocol[REPOSITION_TIME];
      showHand = 0;
      showVRef = 0;
    state WaitAtRefPointP/
      event_code = E_WAIT_AT_REF;
      tone = 1;
      tickCount = Trial_Protocol[REF_HOLD_TIME] ;
      showHand = 0;
      showVRef = (Trial_Protocol[TRIAL_TYPE] > 2); //show if VP trial
      showPRef = 3;
    state WaitBeforeReport/
      showVRef = 0;
      showPRef = 0;
      showHand = 0;
      tone = 0;
    state MoveBack2start_seg2/
      // The hand is in the reference point so start respositioning it by incrementing t_step
      event_code = E_ROBOT_RETURN_TO_START;
      showVRef = 0;
      //showHand = 0
      //refxy[2] = Target_Table[refPointNum][2]; //change back (in the VP cases it gets changed sometimes)
      curhandxy[1] = CurrHandPos[1];
      curhandxy[2] = CurrHandPos[2];
      //start is refxy
      cpRows[1] = Trial_Protocol[CP3]; //CP1
      cpRows[2] = Trial_Protocol[CP4];
      cpRows[3] = -1;
      cpRows[4] = -1;//CP4
      endhandxy[1] = startxy[1];
      endhandxy[2] = startxy[2];
      segcount = 1; //move along curvy bezier curve
      t_step = 0;
      //increment t_step on each clock cycle
      during:
      on e_clk: t_step = t_step + (1.0/ (Trial_Protocol[REPOSITION_TIME]));
    state ReleaseHandHold/
      event_code = E_HOLD_POS;
      tickCount = Trial_Protocol[WAIT_REPORT_TIME];
      enable_controller=0;
    state Report/
      event_code = E_GO_CUE;
      tone = 2; // MI some tone to indicate reporting??
      showStartTgt = 0;
      tickCount = Trial_Protocol[REPORT_TIME];
      t = 0;
      //during:
      //on e_clk: t = t+1;
    state WaitHandInTgt/ [commented out]
      tickCount = Trial_Protocol[WAIT_REPORT_TIME] ;
    state HandMoving/
      event_code = E_HAND_MOVING;
      tone = 0;
      during:
      on e_clk: t = t+1;
    state TooSlow/
      event_code = E_MOVE_TIMEOUT;
      tone = 3;  //error tone
      showSlowMsg = 1; //display Too Slow message
      Repeat_Trial_Flag = 1; //assert repeat trial flag?
      //turn on the position controller to catch the hand
      response[1] = -1; //report xy position
      response[2] = -1;
      curhandxy[1] = CurrHandPos[1]; //report xy position
      curhandxy[2] = CurrHandPos[2];
      segcount = 3;
      enable_controller = 1;
    state HandStill/
      during:
      on e_clk: t = t+1;
    state EndOfTrial1/
      //record what ref point was used, reset values
      event_code = E_END_TRIAL;
      showStartTgt = 0;
    state Feedback/
      //allow participant to try to replicate distance from origin (1600 ms)
      event_code = E_RESPONSE_RECORDED;
      tone = 2;
      curhandxy[1] = CurrHandPos[1]; //report xy position
      curhandxy[2] = CurrHandPos[2];
      segcount = 3;
      enable_controller = 1;
      response[1] = CurrHandPos[1]; //report xy position
      response[2] = CurrHandPos[2];
      showHand = (Trial_Protocol[TRIAL_TYPE]< 3); // only show if not VP
      showVRef = (Trial_Protocol[TRIAL_TYPE] == 1); // show if V trial
      showPRef = (Trial_Protocol[TRIAL_TYPE] == 2); // show if P trial
      tickCount = 1000;
    MoveToStart -> InitPauseTrial1 [order 2] : [cuetarget_state==5]
        | // analogous with trial type
    InitPauseTrial1 -> EndOfTrial1 : [taskbtn==4]
    MoveToStart -> PauseStart [order 1] : // t done incrementing
        | [(t_step >= 1)]/  //&& HandInTarget(startNum)
        | t_step = 1;
    PauseStart -> PauseStart2 : [after(tickCount,e_clk)  && (HandInTarget[startNum] == 1)]
    PauseStart2 -> waitBeforeReport1 : [after(tickCount,e_clk)] /
        | cuetarget_state=0;
    waitBeforeReport1 -> HoldStart [order 1] : //trial type is Visual
        | [(Trial_Protocol[TRIAL_TYPE] == 1)]
    HoldStart -> ShowReference : after(tickCount,e_clk)
    waitBeforeReport1 -> Move2reference_seg1P [order 2] : // if trial type is P or VP
        | [(Trial_Protocol[TRIAL_TYPE] > 1)]
    ShowReference -> BlankScreen : after(tickCount,e_clk)
    Move2reference_seg1P -> WaitAtRefPointP : // t done incrementing
        | [(t_step >= 1)]/
        | t_step = 1;
    WaitAtRefPointP -> MoveBack2start_seg2 : [after(tickCount,e_clk)]/ //&& (HandInTarget[refPointNum] == 1)
    BlankScreen -> WaitBeforeReport : after(tickCount,e_clk)
    MoveBack2start_seg2 -> WaitBeforeReport : // t done incrementing
        | [(t_step >= 1)]/
        | t_step = 1;
    WaitBeforeReport -> ReleaseHandHold : after(500,e_clk)
    ReleaseHandHold -> Report : [after(tickCount,e_clk)]/
    WaitHandInTgt -> ReleaseHandHold [commented out] : [HandInTarget[startNum] == 0]
    WaitHandInTgt -> Report [commented out] : // wait in start point
        | after(tickCount,e_clk)
    Report -> HandMoving [order 1] : [HandVelocity > TaskwideParams[K_VEL_MIN]]
    Report -> TooSlow [order 2] : [t >= tickCount]
    HandMoving -> TooSlow [order 2] : [t >= tickCount]
    HandMoving -> HandStill [order 1] : [HandVelocity < TaskwideParams[K_VEL_MIN]]
    HandStill -> HandMoving [order 1] : [HandVelocity > TaskwideParams[K_VEL_MIN]]
    HandStill -> Feedback [order 2] : //hand stopped moving
        | after(500,e_clk)
    TooSlow -> EndOfTrial1
    Feedback -> EndOfTrial1 : after(tickCount,e_clk)
  note: ?
  state Inter_Trial_State/
    //reset the event code, and send the
    //e_Trial_End Stateflow event to indicate that the trial is over.
    event_code = 0;
    tickCount = Trial_Protocol[DELAY_POST_TRIAL_COL]
    showSlowMsg = 0;
    e_Trial_End;
  state RobotRampDown1/
    enable_controller = 0;
    ramp_time = 2000;
  (default) -> Initialize1
  Initialize1 -> MoveToStart : after(tickCount,e_clk)/
  Inter_Trial_State -> MoveToStart : after(1000,e_clk)
  EndOfTrial1 -> Inter_Trial_State : after(100, e_clk)
  RobotRampDown1 -> Inter_Trial_State : after(ramp_time,e_clk)
  Task1 -> RobotRampDown1 : e_ExitTrialNow/
      | tickCount = 1;
      | // e_ExitTrialNow event occurs if the
      | // Dex pause is pressed by the operator
  data: elapsed_time local double; event_code output uint16 [0..] =0; response output double size=[1 2]; enable_controller output double; tickCount local double; Trial_Protocol input double; HandInTarget input double size=[64 1]; TaskwideParams input double; HandVelocity input double; ramp_time local double; t_step output double size=1; curhandxy output double size=[1 2]; segcount output double size=1; cpRows output double size=[1 5]; endhandxy output double size=[1 2]; startNum output double size=1; showStartTgt output double; refPointNum output double size=1; showVRef output double size=1; showPRef output double; Voffset output double size=[1 2]; Poffset output double size=[1 2]; Target_Table input double size=[64 25]; tone output double size=1; showSlowMsg output double; CurrHandPos input double size=[1 2]; refxy local double size=[1 2]; showHand output double size=1; Repeat_Trial_Flag output boolean; startxy local double size=[1 2]; t local double; cuetarget_row output double; cuetarget_state output double; CueType output double; taskbtn input double; jitter_x output double; jitter_y output double; startTarget_ref local double
  events: e_clk input RISING_EDGE_EVENT; e_ExitTrialNow input EITHER_EDGE_EVENT; e_Trial_End output EITHER_EDGE_EVENT

== matlab function CML_Static_Sensory_Weighting/BezierCurve/Bezier_fnc ==
  data: curxy input size=[1 2]; segCount input; desiredPos output size=[1 2]; VCODE input; VCODE_mod output; t input; cpRows input size=[1 5]; control_points input; endxy input size=[1 2]; CPS output size=[1 8]
function [desiredPos,VCODE_mod, CPS] = fcn(curxy,segCount,VCODE,t,cpRows,control_points,endxy)
%#codegen

VCODE_mod = VCODE;

%clip t just in case!
if t < 0
    t = 0;
elseif t > 1;
    t = 1;
end

t = t-sin(2*pi*t)/(2*pi);  %use the bell-shaped velocity profile from the trajectory controller




ncps = sum(cpRows > 0); %we will assume control points are filled in sequentially so you have a few valid CPs and then none after that


dPos = [0 0];
cp1 = [0 0];
cp2 = [0 0];
cp3 = [0 0];
cp4 = [0 0];
cp5 = [0 0];
cp6 = [0 0];





if segCount == 1  %seg == 1 takes you from the current hand position to a target via control points

    cp1 = curxy;
    
    if ncps == 0  %linear
    
        %2 point bezier
        cp2 = endxy;
        
        dPos = (1-t)*cp1 + t*cp2;

        
    elseif ncps == 1  %quadratic 
    
        %3 point bezier
        cp2 = [control_points(cpRows(1),1), control_points(cpRows(1),2)]; %CP1X and CP1Y
        cp3 = endxy;
        
        dPos = ((1-t)^2)*cp1 + 2*(1-t)*t*cp2 + (t^2)*cp3;
        
    elseif ncps == 2  %cubic
        
        %4 point bezier
        cp2 = [control_points(cpRows(1),1), control_points(cpRows(1),2)]; %CP1X and CP1Y
        cp3 = [control_points(cpRows(2),1), control_points(cpRows(2),2)]; %CP2X and CP2Y
        cp4 = endxy;
        
        dPos = ((1-t)^3)*cp1 + 3*((1-t)^2)*t*cp2 + 3*(1-t)*(t^2)*cp3 + (t^3)*cp4;
        
    elseif ncps == 3  %quartic

        %5 point bezier
        cp2 = [control_points(cpRows(1),1), control_points(cpRows(1),2)]; %CP1X and CP1Y
        cp3 = [control_points(cpRows(2),1), control_points(cpRows(2),2)]; %CP2X and CP2Y
        cp4 = [control_points(cpRows(3),1), control_points(cpRows(3),2)]; %CP3X and CP3Y
        cp5 = endxy;
        
        dPos = ((1-t)^4)*cp1 + 4*((1-t)^3)*t*cp2 + 6*((1-t)^2)*(t^2)*cp3 + 4*(1-t)*(t^3)*cp4 + (t^4)*cp5;

        
    else%if cps == 4   %quintic
    
        %6 point bezier
        cp2 = [control_points(cpRows(1),1), control_points(cpRows(1),2)]; %CP1X and CP1Y
        cp3 = [control_points(cpRows(2),1), control_points(cpRows(2),2)]; %CP2X and CP2Y
        cp4 = [control_points(cpRows(3),1), control_points(cpRows(3),2)]; %CP3X and CP3Y
        cp5 = [control_points(cpRows(4),1), control_points(cpRows(4),2)]; %CP4X and CP4Y %+startxy(1)-center(1)+startxy(2)-center(2)
        cp6 = endxy;
        
        dPos = ((1-t)^5)*cp1 + 5*t*((1-t)^4)*cp2 + 10*(t^2)*((1-t)^3)*cp3 + 10*(t^3)*((1-t)^2)*cp4 + 5*(t^4)*(1-t)*cp5 + (t^5)*cp6;
        
    end
    
    
elseif segCount == 2  %seg == 2 uses a linear bezier from the current hand position to target
    
    cp1 = curxy;
    cp2 = endxy;
    cp3 = [NaN NaN];
    cp4 = [NaN NaN];
    cp5 = [NaN NaN];
    
    dPos = (1-t)*cp1 + t*cp2;

else %if segCount == 3  %seg == 3 holds the hand where it is currently 
    
    dPos = curxy;
    
end



desiredPos = dPos; %to get to cm
desiredPos = desiredPos/100;

CPS = [cp2 cp3 cp4 cp5];

VCODE_mod(3) = desiredPos(1); %convert to meters
VCODE_mod(4) = desiredPos(2); %convert to meters

== stateflow chart CML_Static_Sensory_Weighting/Subsystem2/Chart ==
  state EnableState/
    state AutoMoveToPos/
      //smoothly creates a trajectory to get the hand to a point eventually
      state MovingToDesiredXY/
        tickCount = TaskwideParams[K_TIME_TO_START];
        state = 11;
        tick = 0;
        during:
        on e_clk: tick++;
        // the trajectory velocity will have a bell shaped profile
        trajectory_shape = tick/tickCount-sin(2*pi*tick/tickCount)/(2*pi);
        virtual_pos[1] = StartPos[1] + (TgtPos[1] - StartPos[1]) * trajectory_shape;
        virtual_pos[2] = StartPos[2] + (TgtPos[2] - StartPos[2]) * trajectory_shape;
      state GetDesiredXY/
        //grab the current desired pos in case it changes
        TgtPos[1] = DesiredPos[1];
        TgtPos[2] = DesiredPos[2];
        StartPos[1] = HandPos[1];
        StartPos[2] = HandPos[2];
        updatepos = 0;
        state = 10;
      state HoldAtDesiredXY/
        //pause until something changes
        state = 12;
        updatepos = 0;
        during:
        on e_clk: updatepos = ( (abs(TgtPos[1]-DesiredPos[1]) > 0.01) || (abs(TgtPos[2]-DesiredPos[2]) > 0.01) )
      GetDesiredXY -> MovingToDesiredXY : after(1, e_clk)
      HoldAtDesiredXY -> GetDesiredXY : [updatepos == 1 && MovOnTraj == 0]
      MovingToDesiredXY -> HoldAtDesiredXY : after(tickCount, e_clk)/
    state MoveAlongTraj/
      //take a step along a trajectory specified externally
      state GetDesiredXY_Traj/
        TgtPos[1] = DesiredPos[1];
        TgtPos[2] = DesiredPos[2];
        StartPos[1] = HandPos[1];
        StartPos[2] = HandPos[2];
        state = 21;
        //movIsSafe = ( (abs(TgtPos[1]-HandPos[1]) < 0.02) || (abs(TgtPos[2]-HandPos[2]) < 0.02) );
        movIsSafe = 1;
      state MovAlongTraj/
        state = 22;
        virtual_pos[1] = DesiredPos[1];
        virtual_pos[2] = DesiredPos[2];
      GetDesiredXY_Traj -> MovAlongTraj [order 2] : [movIsSafe == 1]
      MovAlongTraj -> GetDesiredXY_Traj
    (junction 15) -> GetDesiredXY [order 1] : [MovOnTraj == 0]
    (junction 15) -> GetDesiredXY_Traj [order 2] : [MovOnTraj == 1]
    MoveAlongTraj -> GetDesiredXY : [MovOnTraj == 0]
    GetDesiredXY_Traj -> GetDesiredXY [order 1] : [movIsSafe == 0]
    AutoMoveToPos -> GetDesiredXY_Traj : [MovOnTraj == 1]
  state Init/
    ramp_time = TaskwideParams[K_ROBOT_RAMP_TIME];
    scale_increment = 1/ramp_time;
    force_scale = 0;
    state = 1;
    during:
    CurrHandPos[1] = HandPos[1];
    CurrHandPos[2] = HandPos[2];
  state RampUp/
    //ramp up the force scale to 1
    CurrHandPos[1] = HandPos[1];
    CurrHandPos[2] = HandPos[2];
    virtual_pos[1] = HandPos[1];
    virtual_pos[2] = HandPos[2];
    state = 2;
    force_scale = 0;
    during:
    on e_clk: force_scale += scale_increment;
  state ResetController/
    reset_controller;
  state RampDown/
    //ramp down the force scale to 1
    CurrHandPos[1] = HandPos[1];
    CurrHandPos[2] = HandPos[2];
    virtual_pos[1] = CurrHandPos[1];
    virtual_pos[2] = CurrHandPos[2];
    state = 30
    during:
    on e_clk: force_scale -= scale_increment;
  (default) -> Init
  Init -> ResetController : //if controller becomes enabled
      | [enable_controller == 1]/
      | force_scale = 0;
  ResetController -> RampUp
  RampUp -> (junction 15) [order 2] : [force_scale >= 1]/
      | force_scale = 1;
  RampDown -> Init [order 2] : [force_scale <0]/
      | force_scale = 0;
  RampDown -> RampUp [order 1] : [enable_controller == 1]
      | //if the controller is enabled
  RampUp -> RampDown [order 1] : [enable_controller == 0]
      | //if the controller gets shut off
  EnableState -> RampDown : [enable_controller == 0]
  data: enable_controller input double; DesiredPos input; HandPos input; TaskwideParams input; force_scale output double; virtual_pos output double size=2; tickCount local double; StartPos local double size=2; TgtPos local double size=2; updatepos local boolean; MovOnTraj input double; CurrHandPos local double size=2; ramp_time local double; scale_increment local double; tick local double; trajectory_shape local double; movIsSafe local boolean; pi constant double =3.14159265358979; state output double
  events: e_clk input EITHER_EDGE_EVENT; reset_controller output EITHER_EDGE_EVENT

== matlab function CML_Static_Sensory_Weighting/Subsystem2/MATLAB Function ==
  data: pos input; VCODE_MOD output; VCODE input
function VCODE_MOD = fcn(pos,VCODE)
%#codegen

VCODE_MOD = VCODE;

VCODE_MOD(3) = pos(1);
VCODE_MOD(4) = pos(2);

== matlab function CML_Static_Sensory_Weighting/MakeTargets/Add_Jitter ==
  data: VCODES input; VCODES_jitter output; j_x input; j_y input
function VCODES_jitter = Calc_TargetPos(VCODES, j_x, j_y)
%#codegen

VCODES_jitter = VCODES;
%convert from cm to m
jitter_x = j_x/100;
jitter_y = j_y/100;

for ii=1:size(VCODES_jitter,1) % cycle every vcode target
    VCODES_jitter(ii,3) = VCODES_jitter(ii,3) + jitter_x;  %x dim
    VCODES_jitter(ii,4) = VCODES_jitter(ii,4) + jitter_y;  %y dim
end
